simulink model "TwoLoopModelBasedController"  (R2020b)
settings: Solver=ode4  StartTime=0.0  StopTime=100.0  FixedStep=1e-3  RelTol=1e-3
settings Model: Creator=Ivan Lopez  LastModifiedBy=Ivan Lopez

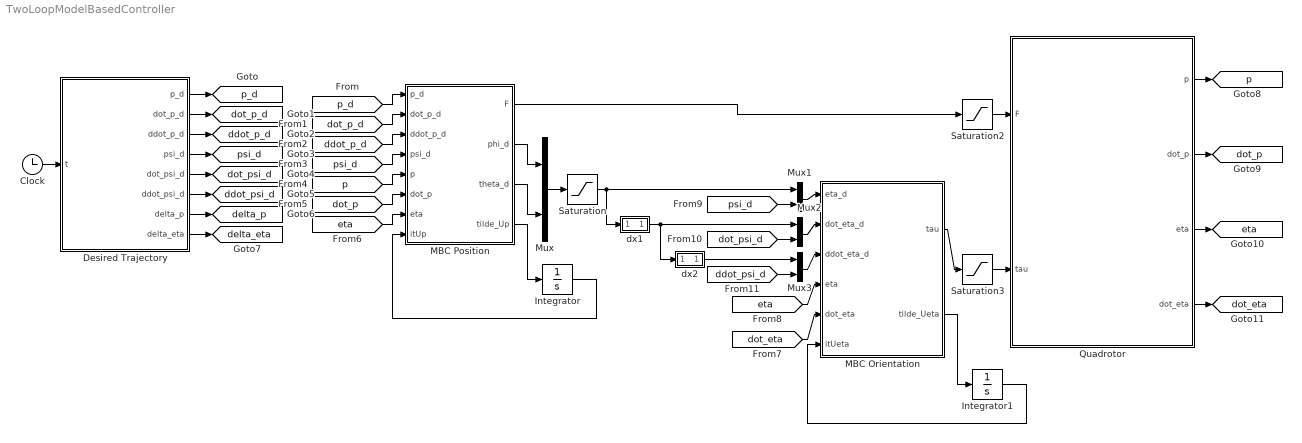
== system TwoLoopModelBasedController ==
  Clock : Clock
  Desired Trajectory : MATLAB Function  TreatAsAtomicUnit=on
  Integrator : Integrator  InitialCondition=[0;0;0]
  Integrator1 : Integrator  InitialCondition=[0;0;0]
  MBC Orientation : MATLAB Function  TreatAsAtomicUnit=on
  MBC Position : MATLAB Function  TreatAsAtomicUnit=on
  Mux{,1..3} (4 alike) : Mux  Inputs=2
  Quadrotor : Subsystem
  Saturation : Saturate  UpperLimit=20*pi/180  LowerLimit=-20*pi/180
  Saturation2 : Saturate  UpperLimit=34.4  LowerLimit=0
  Saturation3 : Saturate  UpperLimit=1.72  LowerLimit=-1.72
  dx1 : Subsystem
  dx2 : Subsystem
  tag scope: ddot_p_d=global, ddot_psi_d=global, delta_eta=global, delta_p=global, dot_eta=global, dot_p=global, dot_p_d=global, dot_psi_d=global, eta=global, p=global, p_d=global, psi_d=global
  wires:
  Clock/1 -> Desired Trajectory/1(t)
  Mux/1 -> Saturation/1
  MBC Position/3(theta_d) -> Mux/2
  MBC Position/2(phi_d) -> Mux/1
  Saturation/1 -> Mux1/1, dx1/1(x)
  Desired Trajectory/1(p_d) -> [p_d]
  Desired Trajectory/3(ddot_p_d) -> [ddot_p_d]
  Desired Trajectory/2(dot_p_d) -> [dot_p_d]
  Desired Trajectory/4(psi_d) -> [psi_d]
  Desired Trajectory/5(dot_psi_d) -> [dot_psi_d]
  Desired Trajectory/6(ddot_psi_d) -> [ddot_psi_d]
  Desired Trajectory/7(delta_p) -> [delta_p]
  Desired Trajectory/8(delta_eta) -> [delta_eta]
  [dot_p_d] -> MBC Position/2(dot_p_d)
  [ddot_p_d] -> MBC Position/3(ddot_p_d)
  [p_d] -> MBC Position/1(p_d)
  [psi_d] -> MBC Position/4(psi_d)
  Quadrotor/1(p) -> [p]
  Quadrotor/2(dot_p) -> [dot_p]
  Quadrotor/3(eta) -> [eta]
  Quadrotor/4(dot_eta) -> [dot_eta]
  [p] -> MBC Position/5(p)
  [dot_p] -> MBC Position/6(dot_p)
  [eta] -> MBC Position/7(eta)
  [dot_eta] -> MBC Orientation/5(dot_eta)
  [eta] -> MBC Orientation/4(eta)
  dx1/1(dx) -> dx2/1(x), Mux2/1
  [psi_d] -> Mux1/2
  [dot_psi_d] -> Mux2/2
  [ddot_psi_d] -> Mux3/2
  dx2/1(dx) -> Mux3/1
  Mux3/1 -> MBC Orientation/3(ddot_eta_d)
  Mux2/1 -> MBC Orientation/2(dot_eta_d)
  Mux1/1 -> MBC Orientation/1(eta_d)
  MBC Position/1(F) -> Saturation2/1
  MBC Orientation/1(tau) -> Saturation3/1
  Saturation3/1 -> Quadrotor/2(tau)
  Saturation2/1 -> Quadrotor/1(F)
  MBC Position/4(tilde_Up) -> Integrator/1
  Integrator/1 -> MBC Position/8(itUp)
  MBC Orientation/2(tilde_Ueta) -> Integrator1/1
  Integrator1/1 -> MBC Orientation/6(itUeta)

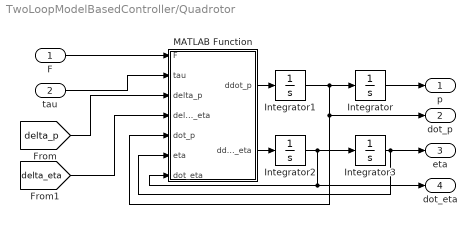
== system TwoLoopModelBasedController/Quadrotor ==
  F : Inport
  tau : Inport  Port=2
  Integrator : Integrator  InitialCondition=[0;0;0.3]  LimitOutput=on  UpperSaturationLimit=[inf;inf;inf]  LowerSaturationLimit=[-inf;-inf;0.3]
  Integrator1 : Integrator  InitialCondition=[0;0;0]
  Integrator2 : Integrator  InitialCondition=[0;0;0]
  Integrator3 : Integrator  InitialCondition=[0;0;0]  LimitOutput=on  UpperSaturationLimit=[pi/2; pi/2; inf]  LowerSaturationLimit=[-pi/2; -pi/2; -inf]
  MATLAB Function : MATLAB Function  TreatAsAtomicUnit=on
  p : Outport
  dot_p : Outport  Port=2
  eta : Outport  Port=3
  dot_eta : Outport  Port=4
  wires:
  [delta_p] -> MATLAB Function/3(delta_p)
  [delta_eta] -> MATLAB Function/4(delta_eta)
  F/1 -> MATLAB Function/1(F)
  Integrator3/1 -> MATLAB Function/6(eta), eta/1
  Integrator1/1 -> dot_p/1, MATLAB Function/5(dot_p), Integrator/1
  MATLAB Function/2(ddot_eta) -> Integrator2/1
  MATLAB Function/1(ddot_p) -> Integrator1/1
  tau/1 -> MATLAB Function/2(tau)
  Integrator2/1 -> Integrator3/1, dot_eta/1, MATLAB Function/7(dot_eta)
  Integrator/1 -> p/1

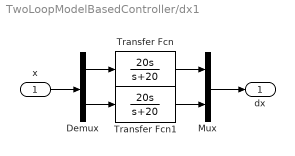
== system TwoLoopModelBasedController/dx1 ==
  x : Inport
  Demux : Demux  Outputs=2
  Mux : Mux  Inputs=2
  Transfer Fcn : TransferFcn  Numerator=[20 0]  Denominator=[1 20]
  Transfer Fcn1 : TransferFcn  Numerator=[20 0]  Denominator=[1 20]
  dx : Outport
  wires:
  Demux/2 -> Transfer Fcn1/1
  Demux/1 -> Transfer Fcn/1
  Transfer Fcn/1 -> Mux/1
  Transfer Fcn1/1 -> Mux/2
  Mux/1 -> dx/1
  x/1 -> Demux/1

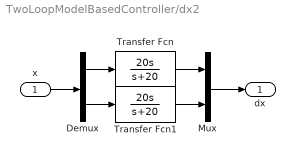
== system TwoLoopModelBasedController/dx2 ==
  x : Inport
  Demux : Demux  Outputs=2
  Mux : Mux  Inputs=2
  Transfer Fcn : TransferFcn  Numerator=[20 0]  Denominator=[1 20]
  Transfer Fcn1 : TransferFcn  Numerator=[20 0]  Denominator=[1 20]
  dx : Outport
  wires:
  x/1 -> Demux/1
  Mux/1 -> dx/1
  Transfer Fcn1/1 -> Mux/2
  Transfer Fcn/1 -> Mux/1
  Demux/1 -> Transfer Fcn/1
  Demux/2 -> Transfer Fcn1/1

== matlab function TwoLoopModelBasedController/MBC Orientation ==
  data: eta_d input; tau output; dot_eta_d input; ddot_eta_d input; eta input; dot_eta input; itUeta input; tilde_Ueta output
function [tau, tilde_Ueta] = fcn(eta_d, dot_eta_d, ddot_eta_d, eta, dot_eta, itUeta)

phi     = eta(1);     theta = eta(2);
dot_phi = dot_eta(1); dot_theta = dot_eta(2);
Ixx = 0.03; Iyy = 0.03; Izz = 0.04;
d_phi = 0.002; d_theta = 0.002; d_psi = 0.004;
I  = diag([Ixx Iyy Izz]);
Dn = diag([d_phi d_theta d_psi]);
%% Gains
K1eta = 2*diag([1 1 1]);
K2eta = 0.001*diag([1 1 1]);
K3eta = 5*diag([1 1 1]);

e_eta     = eta_d - eta;
dot_e_eta = dot_eta_d - dot_eta;

Ueta     = dot_eta_d + K3eta*e_eta;
dot_Ueta = ddot_eta_d + K3eta*dot_e_eta;

tilde_Ueta = Ueta - dot_eta;

W = [1  sin(phi)*tan(theta)  cos(phi)*tan(theta)
     0  cos(phi)             -sin(phi)
     0  sin(phi)/cos(theta)  cos(phi)/cos(theta)];

iW = [1 0         -sin(theta)
      0 cos(phi)  cos(theta)*sin(phi)
      0 -sin(phi) cos(theta)*cos(phi)];
 
dot_W = [0  (cos(phi)*tan(theta))+((sin(phi)*dot_theta)/(cos(theta)^2))                     ((cos(phi)*dot_theta)/(cos(theta)^2))-(sin(phi)*tan(theta)*dot_phi)
         0  -sin(phi)*dot_phi                                                               -cos(phi)*dot_phi
         0  ((cos(phi)*cos(theta)*dot_phi)+(sin(phi)*sin(theta)*dot_theta))/(cos(theta)^2)  ((cos(phi)*sin(theta)*dot_theta)-(sin(phi)*cos(theta)*dot_phi))/(cos(theta)^2)];
  
iWdot_eta = iW*dot_eta;

SiWdot_eta = [0              -iWdot_eta(3)  iWdot_eta(2)
              iWdot_eta(3)   0              -iWdot_eta(1)
              -iWdot_eta(2)  iWdot_eta(1)   0];

M = iW'*I*iW;
C = iW'*(SiWdot_eta*I - I*iW*dot_W)*iW;
tau = W'*(K1eta*tilde_Ueta + K2eta*itUeta + M*dot_Ueta + (C + Dn)*dot_eta);

== matlab function TwoLoopModelBasedController/Quadrotor/MATLAB Function ==
  data: F input; ddot_p output; ddot_eta output; tau input; delta_p input; delta_eta input; dot_p input; eta input; dot_eta input
function [ddot_p, ddot_eta] = fcn(F, tau, delta_p, delta_eta, dot_p, eta, dot_eta)

m  = 1.79;
g  = 9.81;
Ixx = 0.03; Iyy = 0.03; Izz = 0.04;
dx = 0.002; dy = 0.002; dz = 0.004;
d_phi = 0.002; d_theta = 0.002; d_psi = 0.004;
I  = diag([Ixx Iyy Izz]);
Dp = diag([dx dy dz]);
Dn = diag([d_phi d_theta d_psi]);
Vz = [0; 0; 1];

phi     = eta(1);     theta     = eta(2);     psi = eta(3);
dot_phi = dot_eta(1); dot_theta = dot_eta(2);

R = [cos(theta)*cos(psi)  sin(phi)*sin(theta)*cos(psi)-cos(phi)*sin(psi)  cos(phi)*sin(theta)*cos(psi)+sin(phi)*sin(psi)
     cos(theta)*sin(psi)  sin(phi)*sin(theta)*sin(psi)+cos(phi)*cos(psi)  cos(phi)*sin(theta)*sin(psi)-sin(phi)*cos(psi)
     -sin(theta)          sin(phi)*cos(theta)                             cos(phi)*cos(theta)];
 
% W = [1  sin(phi)*tan(theta)  cos(phi)*tan(theta)
%      0  cos(phi)             -sin(phi)
%      0  sin(phi)/cos(theta)  cos(phi)/cos(theta)];

iW = [1 0         -sin(theta)
      0 cos(phi)  cos(theta)*sin(phi)
      0 -sin(phi) cos(theta)*cos(phi)];
 
dot_W = [0  (cos(phi)*tan(theta))+((sin(phi)*dot_theta)/(cos(theta)^2))                     ((cos(phi)*dot_theta)/(cos(theta)^2))-(sin(phi)*tan(theta)*dot_phi)
         0  -sin(phi)*dot_phi                                                               -cos(phi)*dot_phi
         0  ((cos(phi)*cos(theta)*dot_phi)+(sin(phi)*sin(theta)*dot_theta))/(cos(theta)^2)  ((cos(phi)*sin(theta)*dot_theta)-(sin(phi)*cos(theta)*dot_phi))/(cos(theta)^2)];
  
iWdot_eta = iW*dot_eta;

SiWdot_eta = [0              -iWdot_eta(3)  iWdot_eta(2)
              iWdot_eta(3)   0              -iWdot_eta(1)
              -iWdot_eta(2)  iWdot_eta(1)   0];

M = iW'*I*iW;
C = iW'*(SiWdot_eta*I - I*iW*dot_W)*iW;

ddot_p   = (R*Vz*F + delta_p - m*g*Vz - Dp*dot_p)/m;
ddot_eta = M\(iW'*tau + delta_eta - C*dot_eta - Dn*dot_eta);

== matlab function TwoLoopModelBasedController/MBC Position ==
  data: p_d input; F output; dot_p_d input; ddot_p_d input; psi_d input; p input; dot_p input; eta input; phi_d output; theta_d output; itUp input; tilde_Up output
function [F, phi_d, theta_d, tilde_Up] = fcn(p_d, dot_p_d, ddot_p_d, psi_d, p, dot_p, eta, itUp)
m  = 0.7*1.79;
g  = 9.81;
gz = [0; 0; g];
dx = 0.002; dy = 0.002; dz = 0.004;
Dp = diag([dx dy dz]);
phi = eta(1) ; theta = eta(2);

e_p     = p_d - p;
dot_e_p = dot_p_d - dot_p;
%% Position Controller
%Gains
K1p = diag([0.75 0.75 10]); 
K2p = diag([0.004 0.004 1]);
K3p = diag([1.75 1.75 12]);

Up       = dot_p_d + K3p*e_p;
dot_Up   = ddot_p_d + K3p*dot_e_p;
tilde_Up = Up - dot_p;

F_p     = K1p*tilde_Up + K2p*itUp + m*(dot_Up + gz) + Dp*dot_p;
theta_d = atan((F_p(1)*cos(psi_d) + F_p(2)*sin(psi_d))/F_p(3));
phi_d   = atan(cos(theta_d)*(F_p(1)*sin(psi_d) - F_p(2)*cos(psi_d))/F_p(3));
F       = F_p(3)/(cos(phi)*cos(theta));

== matlab function TwoLoopModelBasedController/Desired Trajectory ==
  data: t input; p_d output; dot_p_d output; ddot_p_d output; psi_d output; dot_psi_d output; ddot_psi_d output; delta_p output; delta_eta output
function [p_d, dot_p_d, ddot_p_d, psi_d, dot_psi_d, ddot_psi_d, delta_p, delta_eta] = fcn(t)
z0    = 0.3;
h     = 1.4;
%% Circunferencia
% ampx = 1;
% ampy = 1;
% ampz = 0.1;
% amps = 10*pi/180;
% frecx = 2*pi/5;
% frecy = 2*pi/5;
% frecz = 2*pi/5;
% frecs = 2*pi/5;

%% Lemniscata 1
% 
% ampx = 0.5;
% ampy = 1;
% ampz = 0.4;
% amps = 5*pi/180;
% frecx = 2*pi/4;
% frecy = 2*pi/8;
% frecz = 2*pi/4;
% frecs = 2*pi/4;
% 
% x_d      = ampx*sin(frecx*t);
% dot_x_d  = ampx*frecx*cos(frecx*t);
% ddot_x_d = -ampx*frecx^2*sin(frecx*t);
% 
% y_d      = ampy*cos(frecy*t);
% dot_y_d  = -ampy*frecy*sin(frecy*t);
% ddot_y_d = -ampy*frecy^2*cos(frecy*t);
% 
% if (t>=0 && t<=5)
%     z_d      = h - (h - z0)*exp(-ampz*t^3);
%     dot_z_d  = 3*ampz*t^2*(h - z0)*exp(-ampz*t^3);
%     ddot_z_d = (3*ampz*t^3 - 2)*3*ampz*t*(z0 - h)*exp(-ampz*t^3);
% else
%     z_d      = (h - ampz) + ampz*sin(frecz*t);
%     dot_z_d  = ampz*frecz*cos(frecz*t);
%     ddot_z_d = -ampz*frecz^2*sin(frecz*t);
% end
% 
% psi_d      = [amps*sin(frecs*t)
%               amps*frecs*cos(frecs*t)
%              -amps*frecs^2*sin(frecs*t)];
%        
% p_d      = [x_d; y_d; z_d];
% dot_p_d  = [dot_x_d; dot_y_d; dot_z_d];
% ddot_p_d = [ddot_x_d; ddot_y_d; ddot_z_d];

%% Lemniscata 2 (Experimento)

ampx = 0.5;
ampy = 1;
frecx = 2*pi/4;
frecy = 2*pi/8;
frecz = 2*pi/4;

x_d      = ampx*sin(frecx*t);
dot_x_d  = ampx*frecx*cos(frecx*t);
ddot_x_d = -ampx*frecx^2*sin(frecx*t);

y_d      = ampy*cos(frecy*t);
dot_y_d  = -ampy*frecy*sin(frecy*t);
ddot_y_d = -ampy*frecy^2*cos(frecy*t);

if (t>=0 && t<=5)
    z_d      = 1 - 0.7*exp(-0.1*t^3);
    dot_z_d  = 0.3*t^2*0.7*exp(-0.1*t^3);
    ddot_z_d = 0.3*0.7*(-0.1*3*exp(-0.1*t^3)*t^4 + 2*exp(-0.1*t^3)*t);
else
    z_d      = 1;
    dot_z_d  = 0;
    ddot_z_d = 0;
end

psi_d      = 0;
dot_psi_d  = 0;
ddot_psi_d = 0;
       
p_d      = [x_d; y_d; z_d];
dot_p_d  = [dot_x_d; dot_y_d; dot_z_d];
ddot_p_d = [ddot_x_d; ddot_y_d; ddot_z_d];

%% Disturbances
if (t>=60)
    delta_p = [0.5*sin(2*frecx*t)
               0.5*cos(2*frecy*t)
               0.5*sin(2*frecz*t)];

    d_eta = 0.045*sin(2.5*pi*t-3) + 0.09*sin(2*pi*t-7) + 0.135*sin(0.5*pi*t-9.5) + 0.09*sin(0.3*pi*t) + 0.054*sin(0.15*pi*t+4.5) + 0.045*sin(0.05*pi*t+2) + 0.135*sin(0.01*pi*t+3) + 0.225;
    delta_eta = [d_eta; d_eta; d_eta];
else
    delta_p = [0;0;0];
    delta_eta = [0;0;0];
end
